simulink model "EKF_2020b"  (R2023b)
settings: Solver=FixedStepDiscrete  StartTime=0.0  StopTime=1  FixedStep=Auto  RelTol=1e-4
InitFcn:
  | Ls = 0.0014
  | r = 0.6;
  | T = 0.00001;
  | ke = 0.0354;
model workspace (MAT data in the model file):
  f = Simulink.Signal
  f.DataType = 'single'
  f.Dimensions = 1
  f.DimensionsMode = 'auto'
  f.Complexity = 'real'
  f.SampleTime = -1
  f.SamplingMode = 'auto'
  f.InitialValue = '0.1827'
libraries: slpidlib x2, spsDCVoltageSourceLib x1, spsPermanentMagnetSynchronousMachineLib x1, simulink x1, spsUniversalBridgeLib x1, sps_lib x1
settings Model: SimulationMode=accelerator  Creator=kongbo  LastModifiedBy=13571
settings SolverCC: AutoInsertRateTranBlk=on
settings OptimizationCC: LifeSpan=inf
settings DebuggingCC: MultiTaskRateTransMsg=warning  UnconnectedInputMsg=warning  UnconnectedOutputMsg=warning  UnconnectedLineMsg=warning  SFExecutionAtInitializationDiag=none  ArithmeticOperatorsInVariantConditions=warning
settings ModelReferenceCC: EnableRefExpFcnMdlSchedulingChecks=on
settings SFSimCC: CustomCodeUndefinedFunction=UseInterfaceOnly
settings RTWCC: DLArmComputeVersion=19.05
settings CodeAppCC: StateflowObjectComments=on

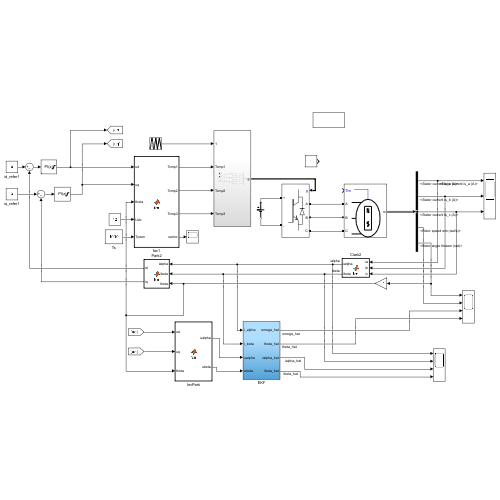
[thumbnail: Simulink's stored preview of the top-level diagram]
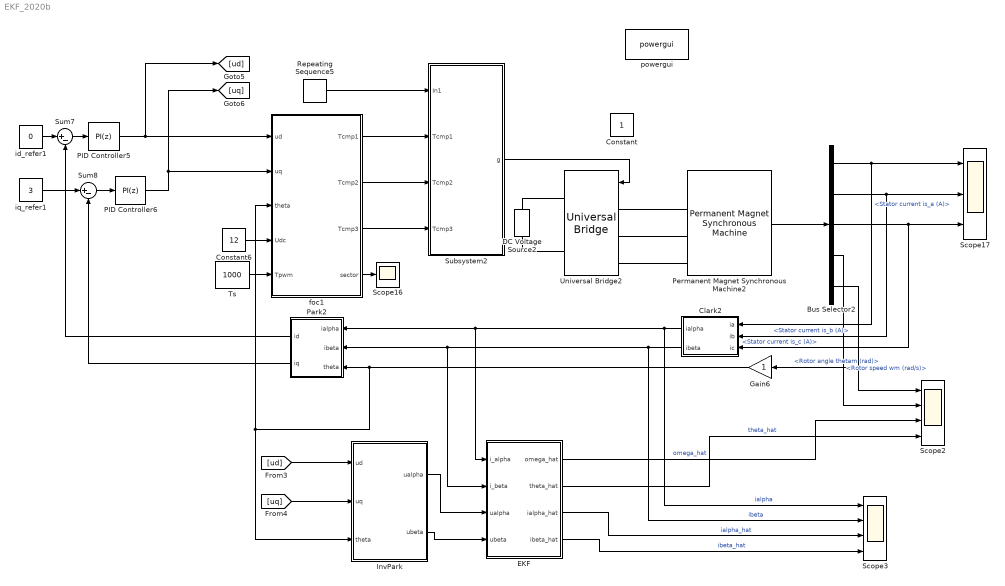
== system EKF_2020b ==
  Bus Selector2 : BusSelector  OutputSignals=Stator current is_a (A),Stator current is_b (A),Stator current is_c (A),Rotor speed wm (rad/s),Rotor angle thetam (rad)
  Clark2 : MATLAB Function  TreatAsAtomicUnit=on
  Constant : Constant
  Constant6 : Constant  Value=12
  DC Voltage Source2 : spsDCVoltageSourceLib/DC Voltage Source  Amplitude=12  Measurements=None
  EKF : Subsystem
  Gain6 : Gain
  InvPark : MATLAB Function  TreatAsAtomicUnit=on
  PID Controller5 : slpidlib/PID Controller  Controller=PI  Form=Parallel  TimeDomain=Discrete-time  UseExternalTs=off  SampleTime=-1  IntegratorMethod=Forward Euler  FilterMethod=Forward Euler  ControllerParametersSource=internal  P=3.6  I=1600  UseKiTs=off  D=0  N=100  UseFilter=on  TunerSelectOption=Transfer Function Based (PID Tuner App)  InitialConditionSource=internal  InitialConditionForIntegrator=0  InitialConditionForFilter=0  DifferentiatorICPrevScaledInput=0  ExternalReset=none  TrackingMode=off  Kt=1  LimitOutput=on  SatLimitsSource=internal  UpperSaturationLimit=12  LowerSaturationLimit=-12  LinearizeAsGain=on  AntiWindupMode=none  Kb=1  LimitIntegrator=off  UpperIntegratorSaturationLimit=inf  LowerIntegratorSaturationLimit=-inf  POutMin=[]  POutMax=[]  IOutMin=[]  IOutMax=[]  DOutMin=[]  DOutMax=[]  NOutMin=[]  NOutMax=[]  SumOutMin=[]  SumOutMax=[]  SaturationOutMin=[]  SaturationOutMax=[]  PParamMin=[]  PParamMax=[]  IParamMin=[]  IParamMax=[]  DParamMin=[]  DParamMax=[]  NParamMin=[]  NParamMax=[]  KbParamMin=[]  KbParamMax=[]  KtParamMin=[]  KtParamMax=[]  KbOutMin=[]  KbOutMax=[]  KtOutMin=[]  KtOutMax=[]  IntegratorOutMin=[]  IntegratorOutMax=[]  FilterOutMin=[]  FilterOutMax=[]  SumI1OutMin=[]  SumI1OutMax=[]  SumI2OutMin=[]  SumI2OutMax=[]  SumI3OutMin=[]  SumI3OutMax=[]  SumI4OutMin=[]  SumI4OutMax=[]  SumDOutMin=[]  SumDOutMax=[]  DifferentiatorOutMin=[]  DifferentiatorOutMax=[]  FilterDiffOutCoefMin=[]  FilterDiffOutCoefMax=[]  ReciprocalOutMin=[]  ReciprocalOutMax=[]  SumDenOutMin=[]  SumDenOutMax=[]  SumNumOutMin=[]  SumNumOutMax=[]  DivideOutMin=[]  DivideOutMax=[]  UdiffTsProdOutMin=[]  UdiffTsProdOutMax=[]  NTsProdOutMin=[]  NTsProdOutMax=[]  UintegralTsProdOutMin=[]  UintegralTsProdOutMax=[]  UngainTsProdOutMin=[]  UngainTsProdOutMax=[]  ClampingZeroOutDataTypeStr=Inherit: Inherit via back propagation  ClampingZeroOutMin=[]  ClampingZeroOutMax=[]  FilterDenConstantOutDataTypeStr=Inherit: Inherit via back propagation  FilterDenConstantOutMin=[]  FilterDenConstantOutMax=[]  PCopyOutDataTypeStr=Inherit: Inherit via back propagation  PCopyOutMin=[]  PCopyOutMax=[]  NCopyOutDataTypeStr=Inherit: Inherit via back propagation  NCopyOutMin=[]  NCopyOutMax=[]  IntegratorContinuousStateAttributes=''  IntegratorStateMustResolveToSignalObject=off  IntegratorRTWStateStorageClass=Auto  FilterContinuousStateAttributes=''  FilterStateMustResolveToSignalObject=off  FilterRTWStateStorageClass=Auto  ParallelPVariant=InternalParameters  IdealPVariant=Disabled  IVariant=InternalParameters  DVariant=Disabled  IntegratorVariant=Discrete  SatVariant=Enabled  AWVariant=Passthrough  PCopyVariant=Disabled  TRVariant=Disabled  FdbkBlocksVariant=Forward  IdealPFdbkVariant=Disabled  SatFdbkVariant=Disabled  DerivativeFilterVariant=Disabled  NVariant=Disabled  NCopyVariant=Disabled_SignalSpec  FilterICVariant=Disabled  IntegratorICVariant=InternalICs  ExternalResetVariant=Disabled  TRSumVariant=Passthrough  SumFdbkVariant=Disabled  SumVariant=Sum_PI  TsampFilterVariant=InternalTs  TsampNgainVariant=Passthrough  TsampIntegralVariant=Disabled_SignalSpec  ExternalSaturationOutDataTypeStr=Inherit: Same as second input
  PID Controller6 : slpidlib/PID Controller  Controller=PI  Form=Parallel  TimeDomain=Discrete-time  UseExternalTs=off  SampleTime=-1  IntegratorMethod=Forward Euler  FilterMethod=Forward Euler  ControllerParametersSource=internal  P=3.6  I=1600  UseKiTs=off  D=0  N=100  UseFilter=on  TunerSelectOption=Transfer Function Based (PID Tuner App)  InitialConditionSource=internal  InitialConditionForIntegrator=0  InitialConditionForFilter=0  DifferentiatorICPrevScaledInput=0  ExternalReset=none  TrackingMode=off  Kt=1  LimitOutput=on  SatLimitsSource=internal  UpperSaturationLimit=12  LowerSaturationLimit=-12  LinearizeAsGain=on  AntiWindupMode=none  Kb=1  LimitIntegrator=off  UpperIntegratorSaturationLimit=inf  LowerIntegratorSaturationLimit=-inf  POutMin=[]  POutMax=[]  IOutMin=[]  IOutMax=[]  DOutMin=[]  DOutMax=[]  NOutMin=[]  NOutMax=[]  SumOutMin=[]  SumOutMax=[]  SaturationOutMin=[]  SaturationOutMax=[]  PParamMin=[]  PParamMax=[]  IParamMin=[]  IParamMax=[]  DParamMin=[]  DParamMax=[]  NParamMin=[]  NParamMax=[]  KbParamMin=[]  KbParamMax=[]  KtParamMin=[]  KtParamMax=[]  KbOutMin=[]  KbOutMax=[]  KtOutMin=[]  KtOutMax=[]  IntegratorOutMin=[]  IntegratorOutMax=[]  FilterOutMin=[]  FilterOutMax=[]  SumI1OutMin=[]  SumI1OutMax=[]  SumI2OutMin=[]  SumI2OutMax=[]  SumI3OutMin=[]  SumI3OutMax=[]  SumI4OutMin=[]  SumI4OutMax=[]  SumDOutMin=[]  SumDOutMax=[]  DifferentiatorOutMin=[]  DifferentiatorOutMax=[]  FilterDiffOutCoefMin=[]  FilterDiffOutCoefMax=[]  ReciprocalOutMin=[]  ReciprocalOutMax=[]  SumDenOutMin=[]  SumDenOutMax=[]  SumNumOutMin=[]  SumNumOutMax=[]  DivideOutMin=[]  DivideOutMax=[]  UdiffTsProdOutMin=[]  UdiffTsProdOutMax=[]  NTsProdOutMin=[]  NTsProdOutMax=[]  UintegralTsProdOutMin=[]  UintegralTsProdOutMax=[]  UngainTsProdOutMin=[]  UngainTsProdOutMax=[]  ClampingZeroOutDataTypeStr=Inherit: Inherit via back propagation  ClampingZeroOutMin=[]  ClampingZeroOutMax=[]  FilterDenConstantOutDataTypeStr=Inherit: Inherit via back propagation  FilterDenConstantOutMin=[]  FilterDenConstantOutMax=[]  PCopyOutDataTypeStr=Inherit: Inherit via back propagation  PCopyOutMin=[]  PCopyOutMax=[]  NCopyOutDataTypeStr=Inherit: Inherit via back propagation  NCopyOutMin=[]  NCopyOutMax=[]  IntegratorContinuousStateAttributes=''  IntegratorStateMustResolveToSignalObject=off  IntegratorRTWStateStorageClass=Auto  FilterContinuousStateAttributes=''  FilterStateMustResolveToSignalObject=off  FilterRTWStateStorageClass=Auto  ParallelPVariant=InternalParameters  IdealPVariant=Disabled  IVariant=InternalParameters  DVariant=Disabled  IntegratorVariant=Discrete  SatVariant=Enabled  AWVariant=Passthrough  PCopyVariant=Disabled  TRVariant=Disabled  FdbkBlocksVariant=Forward  IdealPFdbkVariant=Disabled  SatFdbkVariant=Disabled  DerivativeFilterVariant=Disabled  NVariant=Disabled  NCopyVariant=Disabled_SignalSpec  FilterICVariant=Disabled  IntegratorICVariant=InternalICs  ExternalResetVariant=Disabled  TRSumVariant=Passthrough  SumFdbkVariant=Disabled  SumVariant=Sum_PI  TsampFilterVariant=InternalTs  TsampNgainVariant=Passthrough  TsampIntegralVariant=Disabled_SignalSpec  ExternalSaturationOutDataTypeStr=Inherit: Same as second input
  Park2 : MATLAB Function  TreatAsAtomicUnit=on
  Permanent Magnet Synchronous Machine2 : spsPermanentMagnetSynchronousMachineLib/Permanent Magnet Synchronous Machine  NbPhases=3  FluxDistribution=Sinusoidal  RotorType=Round  MechanicalLoad=Torque Tm  PresetModel=No  ShowDetailedParameters=on  MeasurementBus=off  Resistance=0.6  Inductance=8.5e-3  dqInductances=[5.25e-3 12e-3]  La=1.4e-3  MachineConstant=Flux linkage established by magnets (V.s)  Flux=0.034182  VoltageCst=6.1999  TorqueCst=0.051273  Flat=120  Mechanical=[1.1e-5 1e-3 1 0.02]  PolePairs=4  InitialConditions=[0,0, 0,0]  InitialConditions5ph=[0 0 0 0 0 0]  RefAngle=Aligned with phase A axis (original Park)  IterativeDiscreteModel=Trapezoidal non iterative  TsBlock=-1  TsPowergui=0
  Repeating Sequence5 : simulink/Sources/Repeating Sequence  rep_seq_t=[0 0.0005 0.001]  rep_seq_y=[0 500 0]
  Scope16 : Scope
  Scope17 : Scope  NumInputPorts=3
  Scope2 : Scope  NumInputPorts=4
  Scope3 : Scope  NumInputPorts=4
  Subsystem2 : Subsystem
  Sum7 : Sum  Inputs=|+-
  Sum8 : Sum  Inputs=|+-
  Ts : Constant  Value=1000  OutDataTypeStr=single
  Universal Bridge2 : spsUniversalBridgeLib/Universal Bridge  Arms=3  SnubberResistance=1e5  SnubberCapacitance=inf  Device=IGBT / Diodes  Ron=1e-3  Lon=0  ForwardVoltages="[  0  0  ]"  ForwardVoltage=0  GTOparameters=[ 10e-6 , 20e-6 ]  IGBTparameters=[ 1e-6 , 2e-6 ]  Measurements=None  Measurements_2=None  converterType=Rectifier
  foc1 : MATLAB Function  TreatAsAtomicUnit=on
  id_refer1 : Constant  Value=0
  iq_refer1 : Constant  Value=3
  powergui : sps_lib/powergui  Priority=1  SimulationMode=Discrete  SampleTime=1e-5  frequency=60  Iterations=50  frequencyindice=0  Pbase=100e6  ErrMax=1e-4  UnitsV=kV  UnitsW=MW  buscounter=0  FunctionMessages=off  echomessages=off  EnableUseOfTLC=off  CurrentSourceSwitches=off  DisableSnubberDevices=off  DisableRonSwitches=off  DisableVfSwitches=off  DisplayEquations=off  AutomaticDiscreteSolvers=off  SolverType=Tustin/Backward Euler (TBE)  Interpol=off  ExternalGateDelay=off  methode=off  Ts=100  x0status=blocks  SPID=on  SwTol=0  HookPort=off  NonlinearTolerance=1e-4  nMaxIteration=100  ContinueOnMaxIteration=off  RestoreLinks=warning  ResistiveCurrentMeasurement=off  Frange=[0:2:500]  Ylog=off  Xlog=on  ShowGrid=off  save=off  variable=ZData  structure=0  ZoomFFT=off  StartTime=0.0  cycles=1  DisplayStyle=1  fundamental=60  FreqAxis=off  MaxFrequency=1000  frequencyindicesteady=1  RmsSteady=1  display=off
  wires:
  Repeating Sequence5/1 -> Subsystem2/1(In1)
  Ts/1 -> foc1/5(Tpwm)
  foc1/3(Tcmp3) -> Subsystem2/4(Tcmp3)
  foc1/2(Tcmp2) -> Subsystem2/3(Tcmp2)
  Constant6/1 -> foc1/4(Udc)
  foc1/1(Tcmp1) -> Subsystem2/2(Tcmp1)
  foc1/4(sector) -> Scope16/1
  Subsystem2/1(g) -> Universal Bridge2/1
  Permanent Magnet Synchronous Machine2/1 -> Bus Selector2/1
  Bus Selector2/1 -> Clark2/1(ia), Scope17/1  "<Stator current is_a (A)>"
  Bus Selector2/2 -> Clark2/2(ib), Scope17/2  "<Stator current is_b (A)>"
  Bus Selector2/3 -> Clark2/3(ic), Scope17/3  "<Stator current is_c (A)>"
  Bus Selector2/5 -> Gain6/1, Scope2/1  "<Rotor angle thetam (rad)>"
  Clark2/1(ialpha) -> EKF/1(i_alpha), Park2/1(ialpha), Scope3/1  "ialpha"
  Clark2/2(ibeta) -> EKF/2(i_beta), Park2/2(ibeta), Scope3/2  "ibeta"
  Sum7/1 -> PID Controller5/1
  Sum8/1 -> PID Controller6/1
  Bus Selector2/4 -> Scope2/2  "<Rotor speed wm (rad/s)>"
  id_refer1/1 -> Sum7/1
  iq_refer1/1 -> Sum8/1
  PID Controller6/1 -> foc1/2(uq), [uq]
  [uq] -> InvPark/2(uq)
  [ud] -> InvPark/1(ud)
  InvPark/2(ubeta) -> EKF/4(ubeta)
  InvPark/1(ualpha) -> EKF/3(ualpha)
  PID Controller5/1 -> foc1/1(ud), [ud]
  EKF/4(ibeta_hat) -> Scope3/4  "ibeta_hat"
  EKF/3(ialpha_hat) -> Scope3/3  "ialpha_hat"
  EKF/2(theta_hat) -> Scope2/4  "theta_hat"
  Gain6/1 -> foc1/3(theta), InvPark/3(theta), Park2/3(theta)
  Park2/2(iq) -> Sum8/2
  Park2/1(id) -> Sum7/2
  EKF/1(omega_hat) -> Scope2/3  "omega_hat"
  connections:
  DC Voltage Source2/LConn1 -- Universal Bridge2/RConn2
  DC Voltage Source2/RConn1 -- Universal Bridge2/RConn1
  Universal Bridge2/LConn1 -- Permanent Magnet Synchronous Machine2/LConn1
  Universal Bridge2/LConn3 -- Permanent Magnet Synchronous Machine2/LConn3
  Universal Bridge2/LConn2 -- Permanent Magnet Synchronous Machine2/LConn2

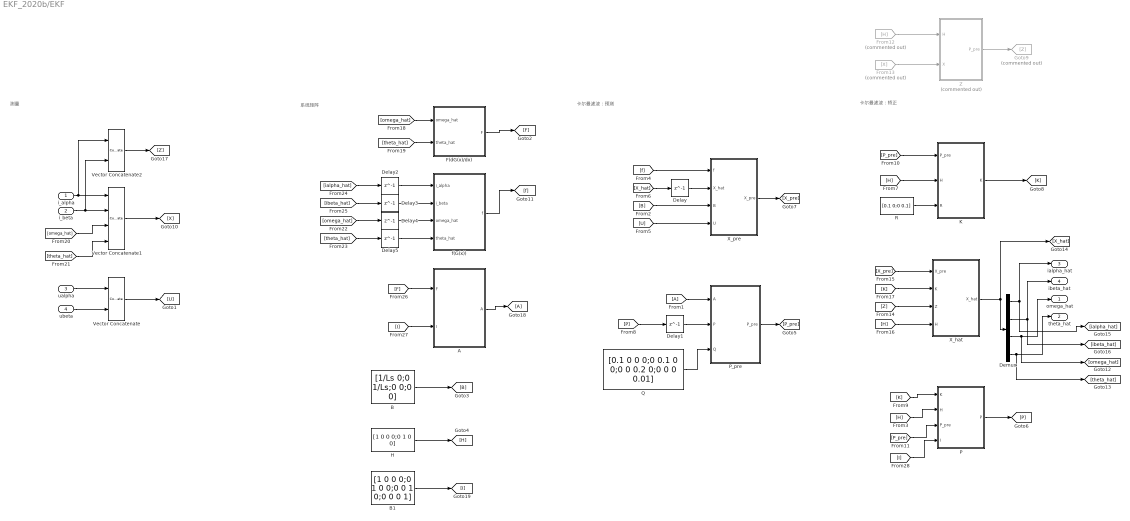
== system EKF_2020b/EKF ==
  note: 卡尔曼滤波：矫正
  note: 测量
  note: 卡尔曼滤波：预测
  note: 系统矩阵
  i_alpha : Inport
  i_beta : Inport  Port=2
  ualpha : Inport  Port=3
  ubeta : Inport  Port=4
  A : Subsystem
  B : Constant  Value=[1/Ls 0;0 1/Ls;0 0;0 0]
  B1 : Constant  Value=[1 0 0 0;0 1 0 0;0 0 1 0;0 0 0 1]
  Delay{,1..5} (6 alike) : Delay  DelayLength=1  InitialCondition=0
  Demux : Demux
  F(dG(x)/dx) : Subsystem
  From1 : From
  From12 : From  Commented=on  GotoTag=H
  From13 : From  Commented=on  GotoTag=X
  Goto18 : Goto
  Goto9 : Goto  Commented=on  GotoTag=Z
  H : Constant  Value=[1 0 0 0;0 1 0 0]
  K : Subsystem
  P : Subsystem
  P_pre : Subsystem
  Q : Constant  Value=[0.1 0 0 0;0 0.1 0 0;0 0 0.2 0;0 0 0 0.01]
  R : Constant  Value=[0.1 0;0 0.1]
  Vector Concatenate : Concatenate  Mode=Multidimensional array
  Vector Concatenate1 : Concatenate  NumInputs=4  Mode=Multidimensional array
  Vector Concatenate2 : Concatenate  Mode=Multidimensional array
  X_hat : Subsystem
  X_pre : Subsystem
  Z : Subsystem  Commented=on
  f(G(x)) : Subsystem
  omega_hat : Outport
  theta_hat : Outport  Port=2
  ialpha_hat : Outport  Port=3
  ibeta_hat : Outport  Port=4
  wires:
  Q/1 -> P_pre/3(Q)
  ualpha/1 -> Vector Concatenate/1
  Vector Concatenate/1 -> [U]
  From1/1 -> P_pre/1(A)
  P/1(P) -> [P]
  F(dG(x)/dx)/1(F) -> [F]
  [K] -> P/1(K)
  [P] -> Delay1/1
  [X_pre] -> X_hat/1(X_pre)
  Z/1(P_pre) -> Goto9/1
  Demux/1 -> [ialpha_hat], ialpha_hat/1
  [K] -> X_hat/2(K)
  Demux/2 -> [ibeta_hat], ibeta_hat/1
  [H] -> P/2(H)
  X_hat/1(X_hat) -> Demux/1, [X_hat]
  [H] -> K/2(H)
  K/1(K) -> [K]
  From12/1 -> Z/1(H)
  H/1 -> [H]
  B/1 -> [B]
  ubeta/1 -> Vector Concatenate/2
  [X_hat] -> Delay/1
  [B] -> X_pre/3(B)
  [H] -> X_hat/4(H)
  Delay/1 -> X_pre/2(X_hat)
  [P_pre] -> P/3(P_pre)
  R/1 -> K/3(R)
  P_pre/1(P_pre) -> [P_pre]
  [P_pre] -> K/1(P_pre)
  Delay1/1 -> P_pre/2(P)
  Demux/4 -> theta_hat/1, [theta_hat]
  [f] -> X_pre/1(f)
  From13/1 -> Z/2(X)
  [omega_hat] -> F(dG(x)/dx)/1(omega_hat)
  X_pre/1(X_pre) -> [X_pre]
  [Z] -> X_hat/3(Z)
  [theta_hat] -> F(dG(x)/dx)/2(theta_hat)
  i_alpha/1 -> Vector Concatenate2/1, Vector Concatenate1/1
  i_beta/1 -> Vector Concatenate2/2, Vector Concatenate1/2
  Vector Concatenate1/1 -> [X]
  [omega_hat] -> Vector Concatenate1/3
  [theta_hat] -> Vector Concatenate1/4
  [U] -> X_pre/4(U)
  f(G(x))/1(f) -> [f]
  [ialpha_hat] -> Delay2/1
  Delay2/1 -> f(G(x))/1(i_alpha)
  [ibeta_hat] -> Delay3/1
  Delay3/1 -> f(G(x))/2(i_beta)
  [omega_hat] -> Delay4/1
  Delay4/1 -> f(G(x))/3(omega_hat)
  [theta_hat] -> Delay5/1
  Delay5/1 -> f(G(x))/4(theta_hat)
  Vector Concatenate2/1 -> [Z]
  [F] -> A/1(F)
  A/1(A) -> Goto18/1
  Demux/3 -> [omega_hat], omega_hat/1
  B1/1 -> [I]
  [I] -> A/2(I)
  [I] -> P/4(I)

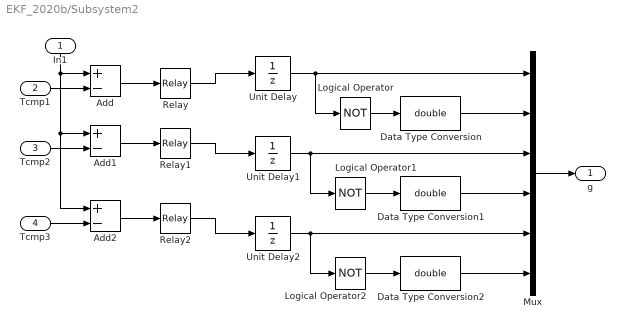
== system EKF_2020b/Subsystem2 ==
  In1 : Inport
  Tcmp1 : Inport  Port=2
  Tcmp2 : Inport  Port=3
  Tcmp3 : Inport  Port=4
  Add : Sum  Inputs=+-
  Add1 : Sum  Inputs=+-
  Add2 : Sum  Inputs=+-
  Data Type Conversion : DataTypeConversion  OutDataTypeStr=double  SaturateOnIntegerOverflow=off  RndMeth=Floor
  Data Type Conversion1 : DataTypeConversion  OutDataTypeStr=double  SaturateOnIntegerOverflow=off  RndMeth=Floor
  Data Type Conversion2 : DataTypeConversion  OutDataTypeStr=double  SaturateOnIntegerOverflow=off  RndMeth=Floor
  Logical Operator : Logic  Operator=NOT  AllPortsSameDT=off  OutDataTypeStr=boolean
  Logical Operator1 : Logic  Operator=NOT  AllPortsSameDT=off  OutDataTypeStr=boolean
  Logical Operator2 : Logic  Operator=NOT  AllPortsSameDT=off  OutDataTypeStr=boolean
  Mux : Mux  Inputs=6
  Relay : Relay  OffSwitchValue=-eps
  Relay1 : Relay  OffSwitchValue=-eps
  Relay2 : Relay  OffSwitchValue=-eps
  Unit Delay : UnitDelay  SampleTime=-1  HasFrameUpgradeWarning=on
  Unit Delay1 : UnitDelay  SampleTime=-1  HasFrameUpgradeWarning=on
  Unit Delay2 : UnitDelay  SampleTime=-1  HasFrameUpgradeWarning=on
  g : Outport
  wires:
  Tcmp3/1 -> Add2/2
  Tcmp2/1 -> Add1/2
  Tcmp1/1 -> Add/2
  Relay2/1 -> Unit Delay2/1
  Relay1/1 -> Unit Delay1/1
  Relay/1 -> Unit Delay/1
  Unit Delay2/1 -> Mux/5, Logical Operator2/1
  Unit Delay1/1 -> Mux/3, Logical Operator1/1
  Unit Delay/1 -> Logical Operator/1, Mux/1
  Mux/1 -> g/1
  Data Type Conversion/1 -> Mux/2
  Data Type Conversion1/1 -> Mux/4
  Data Type Conversion2/1 -> Mux/6
  Logical Operator2/1 -> Data Type Conversion2/1
  Logical Operator1/1 -> Data Type Conversion1/1
  Logical Operator/1 -> Data Type Conversion/1
  Add1/1 -> Relay1/1
  Add2/1 -> Relay2/1
  Add/1 -> Relay/1
  In1/1 -> Add/1, Add2/1, Add1/1

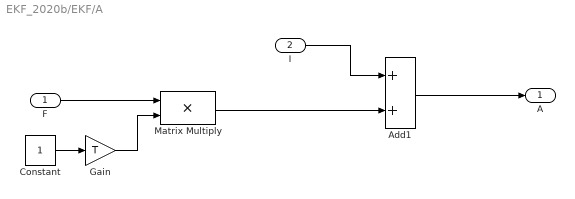
== system EKF_2020b/EKF/A ==
  F : Inport
  I : Inport  Port=2
  Add1 : Sum
  Constant : Constant
  Gain : Gain  Gain=T
  Matrix Multiply : Product
  A : Outport
  wires:
  F/1 -> Matrix Multiply/1
  I/1 -> Add1/1
  Constant/1 -> Gain/1
  Gain/1 -> Matrix Multiply/2
  Matrix Multiply/1 -> Add1/2
  Add1/1 -> A/1

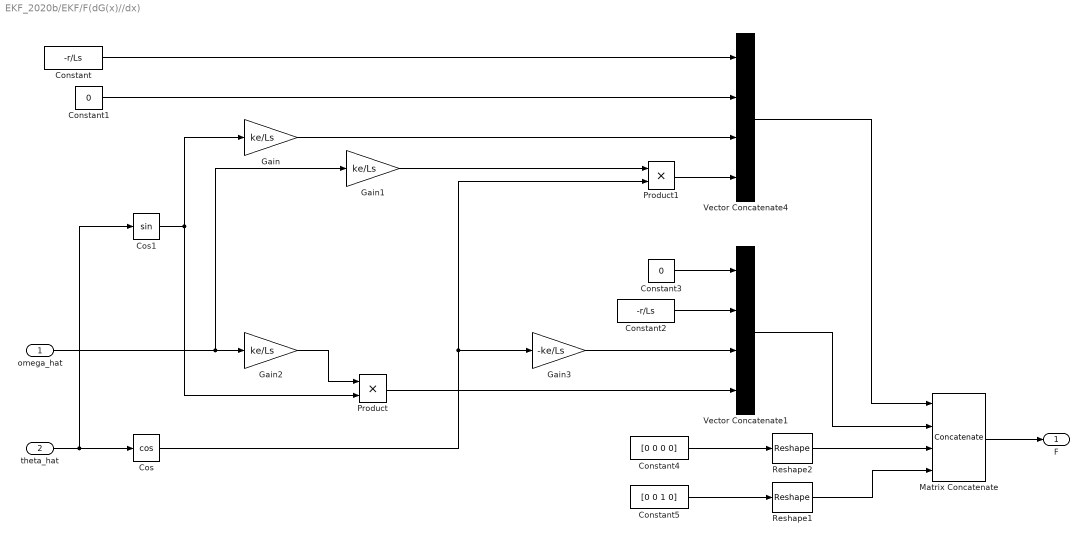
== system EKF_2020b/EKF/F(dG(x)//dx) ==
  omega_hat : Inport
  theta_hat : Inport  Port=2
  Constant : Constant  Value=-r/Ls
  Constant1 : Constant  Value=0
  Constant2 : Constant  Value=-r/Ls
  Constant3 : Constant  Value=0
  Constant4 : Constant  Value=[0 0 0 0]
  Constant5 : Constant  Value=[0 0 1 0]
  Cos : Trigonometry  Operator=cos
  Cos1 : Trigonometry
  Gain : Gain  Gain=ke/Ls
  Gain1 : Gain  Gain=ke/Ls
  Gain2 : Gain  Gain=ke/Ls
  Gain3 : Gain  Gain=-ke/Ls
  Matrix Concatenate : Concatenate  NumInputs=4  Mode=Multidimensional array
  Product : Product
  Product1 : Product
  Reshape1 : Reshape  OutputDimensionality=Row vector (2-D)
  Reshape2 : Reshape  OutputDimensionality=Row vector (2-D)
  Vector Concatenate1 : Concatenate  NumInputs=4  Mode=Multidimensional array  ConcatenateDimension=2
  Vector Concatenate4 : Concatenate  NumInputs=4  Mode=Multidimensional array  ConcatenateDimension=2
  F : Outport
  wires:
  Vector Concatenate4/1 -> Matrix Concatenate/1
  Vector Concatenate1/1 -> Matrix Concatenate/2
  Constant/1 -> Vector Concatenate4/1
  Constant1/1 -> Vector Concatenate4/2
  theta_hat/1 -> Cos1/1, Cos/1
  Cos/1 -> Gain3/1, Product1/2
  Gain/1 -> Vector Concatenate4/3
  omega_hat/1 -> Gain2/1, Gain1/1
  Gain2/1 -> Product/1
  Gain1/1 -> Product1/1
  Product1/1 -> Vector Concatenate4/4
  Constant3/1 -> Vector Concatenate1/1
  Constant2/1 -> Vector Concatenate1/2
  Gain3/1 -> Vector Concatenate1/3
  Product/1 -> Vector Concatenate1/4
  Matrix Concatenate/1 -> F/1
  Constant5/1 -> Reshape1/1
  Constant4/1 -> Reshape2/1
  Reshape2/1 -> Matrix Concatenate/3
  Reshape1/1 -> Matrix Concatenate/4
  Cos1/1 -> Gain/1, Product/2

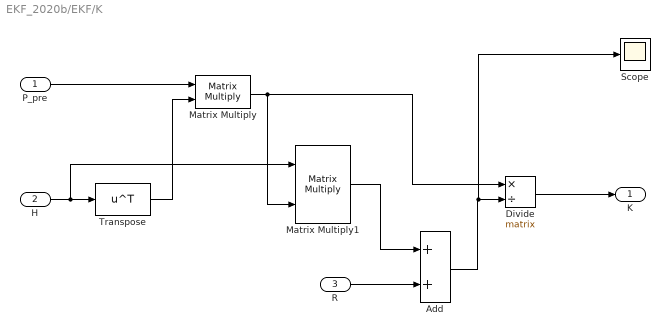
== system EKF_2020b/EKF/K ==
  P_pre : Inport
  H : Inport  Port=2
  R : Inport  Port=3
  Add : Sum
  Divide : Product  Inputs=*/  Multiplication=Matrix(*)
  Matrix Multiply : Product  Multiplication=Matrix(*)
  Matrix Multiply1 : Product  Multiplication=Matrix(*)
  Scope : Scope
  Transpose : Math  Operator=transpose  SignedPower=on
  K : Outport
  wires:
  R/1 -> Add/2
  H/1 -> Matrix Multiply1/1, Transpose/1
  P_pre/1 -> Matrix Multiply/1
  Transpose/1 -> Matrix Multiply/2
  Matrix Multiply1/1 -> Add/1
  Divide/1 -> K/1
  Matrix Multiply/1 -> Divide/1, Matrix Multiply1/2
  Add/1 -> Scope/1, Divide/2

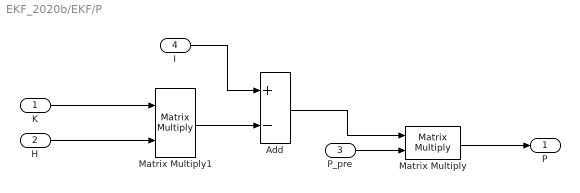
== system EKF_2020b/EKF/P ==
  K : Inport
  H : Inport  Port=2
  P_pre : Inport  Port=3
  I : Inport  Port=4
  Add : Sum  Inputs=+-
  Matrix Multiply : Product  Multiplication=Matrix(*)
  Matrix Multiply1 : Product  Multiplication=Matrix(*)
  P : Outport
  wires:
  I/1 -> Add/1
  K/1 -> Matrix Multiply1/1
  H/1 -> Matrix Multiply1/2
  Matrix Multiply1/1 -> Add/2
  Add/1 -> Matrix Multiply/1
  P_pre/1 -> Matrix Multiply/2
  Matrix Multiply/1 -> P/1

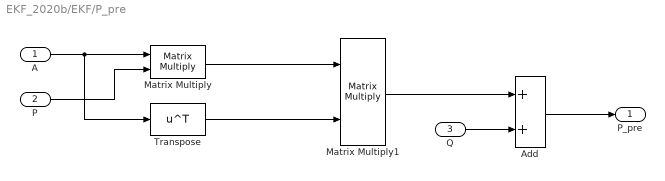
== system EKF_2020b/EKF/P_pre ==
  A : Inport
  P : Inport  Port=2
  Q : Inport  Port=3
  Add : Sum
  Matrix Multiply : Product  Multiplication=Matrix(*)
  Matrix Multiply1 : Product  Multiplication=Matrix(*)
  Transpose : Math  Operator=transpose  SignedPower=on
  P_pre : Outport
  wires:
  A/1 -> Transpose/1, Matrix Multiply/1
  P/1 -> Matrix Multiply/2
  Add/1 -> P_pre/1
  Q/1 -> Add/2
  Matrix Multiply1/1 -> Add/1
  Matrix Multiply/1 -> Matrix Multiply1/1
  Transpose/1 -> Matrix Multiply1/2

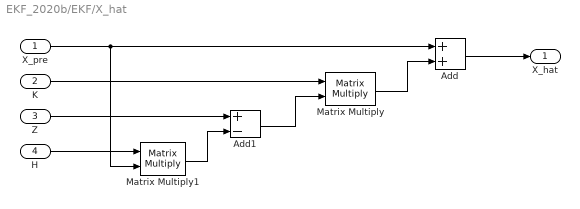
== system EKF_2020b/EKF/X_hat ==
  X_pre : Inport
  K : Inport  Port=2
  Z : Inport  Port=3
  H : Inport  Port=4
  Add : Sum
  Add1 : Sum  Inputs=+-
  Matrix Multiply : Product  Multiplication=Matrix(*)
  Matrix Multiply1 : Product  Multiplication=Matrix(*)
  X_hat : Outport
  wires:
  X_pre/1 -> Matrix Multiply1/2, Add/1
  K/1 -> Matrix Multiply/1
  Z/1 -> Add1/1
  H/1 -> Matrix Multiply1/1
  Matrix Multiply1/1 -> Add1/2
  Add1/1 -> Matrix Multiply/2
  Matrix Multiply/1 -> Add/2
  Add/1 -> X_hat/1

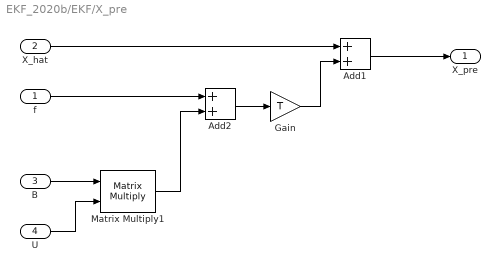
== system EKF_2020b/EKF/X_pre ==
  f : Inport
  X_hat : Inport  Port=2
  B : Inport  Port=3
  U : Inport  Port=4
  Add1 : Sum  OutMin=[0.001]  OutMax=[100]  AccumDataTypeStr=double
  Add2 : Sum  OutMin=[0.001]  OutMax=[100]  AccumDataTypeStr=double
  Gain : Gain  Gain=T
  Matrix Multiply1 : Product  Multiplication=Matrix(*)
  X_pre : Outport
  wires:
  B/1 -> Matrix Multiply1/1
  U/1 -> Matrix Multiply1/2
  X_hat/1 -> Add1/1
  Matrix Multiply1/1 -> Add2/2
  f/1 -> Add2/1
  Add2/1 -> Gain/1
  Gain/1 -> Add1/2
  Add1/1 -> X_pre/1

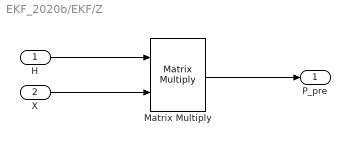
== system EKF_2020b/EKF/Z ==
  H : Inport
  X : Inport  Port=2
  Matrix Multiply : Product  Multiplication=Matrix(*)
  P_pre : Outport
  wires:
  H/1 -> Matrix Multiply/1
  Matrix Multiply/1 -> P_pre/1
  X/1 -> Matrix Multiply/2

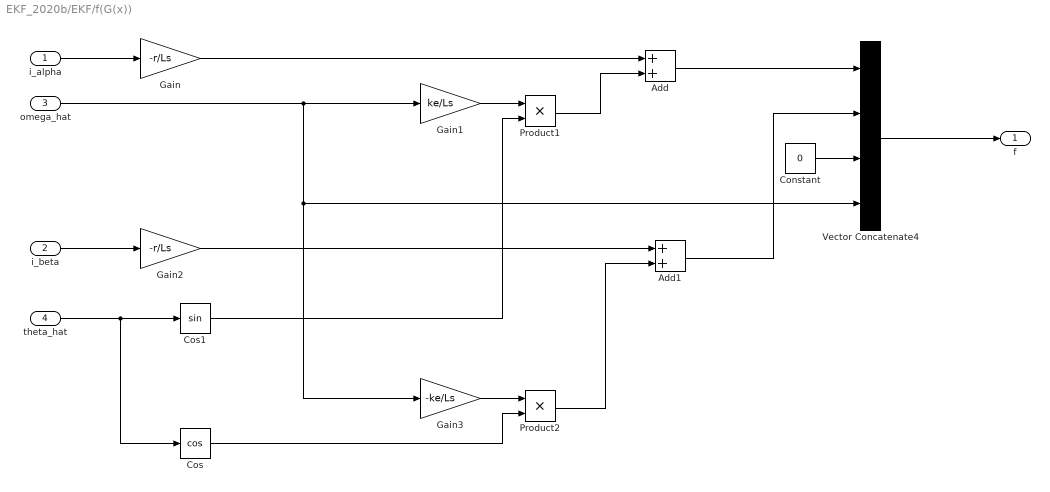
== system EKF_2020b/EKF/f(G(x)) ==
  i_alpha : Inport
  i_beta : Inport  Port=2
  omega_hat : Inport  Port=3
  theta_hat : Inport  Port=4
  Add : Sum
  Add1 : Sum
  Constant : Constant  Value=0
  Cos : Trigonometry  Operator=cos
  Cos1 : Trigonometry
  Gain : Gain  Gain=-r/Ls
  Gain1 : Gain  Gain=ke/Ls
  Gain2 : Gain  Gain=-r/Ls
  Gain3 : Gain  Gain=-ke/Ls
  Product1 : Product
  Product2 : Product
  Vector Concatenate4 : Concatenate  NumInputs=4  Mode=Multidimensional array
  f : Outport
  wires:
  theta_hat/1 -> Cos/1, Cos1/1
  Gain1/1 -> Product1/1
  i_alpha/1 -> Gain/1
  Gain/1 -> Add/1
  omega_hat/1 -> Gain3/1, Vector Concatenate4/4, Gain1/1
  Cos1/1 -> Product1/2
  Product1/1 -> Add/2
  Add/1 -> Vector Concatenate4/1
  Vector Concatenate4/1 -> f/1
  i_beta/1 -> Gain2/1
  Gain2/1 -> Add1/1
  Gain3/1 -> Product2/1
  Cos/1 -> Product2/2
  Product2/1 -> Add1/2
  Add1/1 -> Vector Concatenate4/2
  Constant/1 -> Vector Concatenate4/3

== matlab function EKF_2020b/InvPark ==
  data: ud input; uq input; ualpha output; ubeta output; theta input
function [ualpha,ubeta] = fcn(ud,uq,theta)

ualpha = cos(theta) * ud - sin(theta) * uq;
ubeta  = sin(theta) * ud + cos(theta) * uq;

end

== matlab function EKF_2020b/Clark2 ==
  data: ia input; ialpha output; ib input; ic input; ibeta output
function [ialpha,ibeta] = fcn(ia,ib,ic)
ialpha = ia*2/3-(ib+ic)/3;
ibeta = (ib-ic)*sqrt(3)/3;

== matlab function EKF_2020b/Park2 ==
  data: ialpha input; ibeta input; theta input; id output; iq output
function [id,iq] = fcn(ialpha,ibeta,theta)
id = ialpha*cos(theta)+ibeta*sin(theta);
iq = -ialpha*sin(theta)+ibeta*cos(theta);

== matlab function EKF_2020b/foc1 ==
  data: ud input; Tcmp1 output; uq input; theta input; Udc input; Tpwm input; Tcmp2 output; Tcmp3 output; sector output
function [Tcmp1,Tcmp2,Tcmp3,sector] = fcn(ud,uq,theta,Udc,Tpwm)
Valpha = ud*cos(theta) - uq*sin(theta);
Vbeta = ud*sin(theta) + uq*cos(theta);
%#codegen

sector = single(0);
Tcmp1 = single(0);
Tcmp2 = single(0);
Tcmp3 = single(0);

%========Parameters statement================

    Vref1 = Vbeta;							                   
    Vref2 = (sqrt(3)*Valpha - Vbeta)/2; 				    
    Vref3 = (-sqrt(3)*Valpha - Vbeta)/2;					
   
 %========Sector calculation=================

  if (Vref1>0)
	   sector = single(1);
  end
  if (Vref2>0)
	   sector = sector+single(2);
  end
  if (Vref3>0)
       sector = sector+single(4);
  end

%======== X Y Z calculation===================

X = sqrt(3)*Vbeta*Tpwm/Udc;
Y = Tpwm/Udc*(3/2*Valpha+sqrt(3)/2*Vbeta);
Z = Tpwm/Udc*(-3/2*Valpha+sqrt(3)/2*Vbeta);	         

%==========Duty ratio calculation================
switch (sector)   
    case 1
        T1 = Z; T2 = Y; 
	case 2
        T1 = Y; T2 = -X; 
	case 3
        T1 = -Z; T2 = X; 
	case 4
        T1 = -X; T2 = Z;
	case 5
        T1 = X; T2 = -Y;
    otherwise
        T1 = -Y; T2 = -Z;
end
T = T1+T2;
if T > Tpwm
    T1 = T1/T*Tpwm;
    T2 = T2/T*Tpwm;
else
end
ta = (Tpwm-(T1+T2))/4.0;
tb = ta+T1/2;
tc = tb+T2/2;

%==========Duty ratio calculation================
switch (sector)
    case 1 
        Tcmp1=tb;
        Tcmp2=ta;
        Tcmp3=tc; 
        
    case 2 
        Tcmp1=ta;
        Tcmp2=tc;
        Tcmp3=tb; 
       
    case 3 
        Tcmp1=ta;
        Tcmp2=tb;
        Tcmp3=tc; 
        
    case 4 
        Tcmp1=tc;
        Tcmp2=tb;
        Tcmp3=ta;
        
    case 5 
        Tcmp1=tc;
        Tcmp2=ta;
        Tcmp3=tb;
        
   case 6
       Tcmp1=tb;
       Tcmp2=tc;
       Tcmp3=ta;
end
end
